simulink model "added_test"  (R2020a)
settings: Solver=VariableStepAuto  StartTime=0.0  StopTime=10.0  RelTol=1e-3
settings Model: Creator=kekatos  LastModifiedBy=kekatos

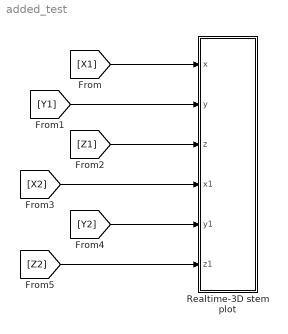
== system added_test ==
  Realtime-3D stem plot : MATLAB Function  TreatAsAtomicUnit=on
  wires:
  [Z1] -> Realtime-3D stem plot/3(z)
  [Y1] -> Realtime-3D stem plot/2(y)
  [Y2] -> Realtime-3D stem plot/5(y1)
  [Z2] -> Realtime-3D stem plot/6(z1)
  [X2] -> Realtime-3D stem plot/4(x1)
  [X1] -> Realtime-3D stem plot/1(x)

== matlab function added_test/Realtime-3D stem plot ==
  data: x input; y input; z input; x1 input; y1 input; z1 input
function  fcn(x, y, z, x1, y1, z1)
figure(1);
hold on; grid on;
coder.extrinsic('stem3');
stem3(x, y, z, 'd', 'k' );
stem3(x1, y1, z1, '+', 'm' );

% coder.extrinsic('plot3');
% plot3(x, y, z, 'd', 'k' );
% plot3(x1, y1, z1, '+', 'm' );

view([45 45]);
